simulink model "Model2"  (R2020a)
settings: Solver=ode4  StartTime=0.0  StopTime=10.0  FixedStep=0.01  RelTol=1e-3
values from neighbouring files (symbols this model uses):
  A = [0 1 0;     0 -0.875 -20;     0 0 -50]    [Zadanie1.m]    (also in Zadanie2.m = [0 1 0 0;     0 -1 0 0;     0 0 0 1;     0 0 0 -1])
  B = [0;      0;      50]    [Zadanie1.m]    (also in Zadanie2.m = [0 0;     1 0;     0 0;     0 1])
  C = eye(4)    [Zadanie2.m]
  Ff = pinv(G)    [Zadanie2.m]
  K = -Km    [Zadanie1.m]
undefined symbols (not defined in the file or in its folder): sigbuilder_block
libraries: robotcorelib x1, simulink x1
settings Model: Creator=grzyb  LastModifiedBy=grzyb

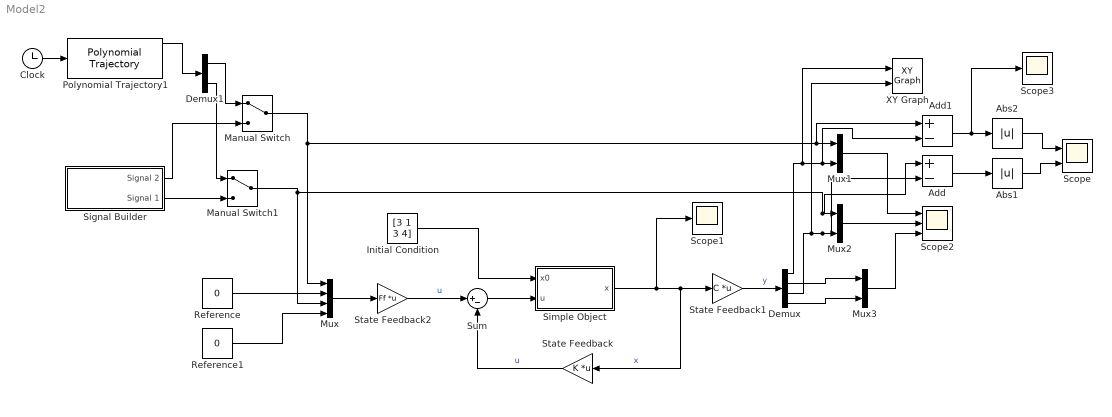
== system Model2 ==
  Abs1 : Abs
  Abs2 : Abs
  Add : Sum  Inputs=+-
  Add1 : Sum  Inputs=+-
  Clock : Clock
  Demux : Demux
  Demux1 : Demux  Outputs=2
  Initial Condition : Constant  Value=[3 1 3 4]
  Manual Switch : ManualSwitch
  Manual Switch1 : ManualSwitch
  Mux : Mux
  Mux1 : Mux  Inputs=2
  Mux2 : Mux  Inputs=2
  Mux3 : Mux  Inputs=2
  Polynomial Trajectory1 : robotcorelib/Polynomial Trajectory  WaypointSource=Internal  Waypoints=[ 0, 2, 1, 3, 0; -1, 3, 1, 4, 4 ]  TimePoints=[ 0, 2, 4, 6, 8 ]  TimeInterval=[ 1, 4 ]  Method=Cubic Polynomial  ParameterSource=Internal  VelocityBoundaryCondition=zeros( 2, 5 )  AccelerationBoundaryCondition=zeros( 2, 5 )  SimulateUsing=Interpreted execution
      settings: SourceProductBaseCode=NV,RO,RR
  Reference : Constant  Value=0
  Reference1 : Constant  Value=0
  Scope : Scope  NumInputPorts=2
  Scope1 : Scope
  Scope2 : Scope  NumInputPorts=3
  Scope3 : Scope
  Signal Builder : Subsystem  Tag=STV Subsys  LoadFcn=sigbuilder_block('load');  StartFcn=sigbuilder_block('start');  StopFcn=sigbuilder_block('stop');  ClipboardFcn=sigbuilder_block('clipboard');  mask(Sigbuilder block){tuvar=[0:10]}
      mask help: Simulink:masks:SigbuilderBlock_MD
      mask init:
      | if ~strcmp(get_param(bdroot(gcbh),'SimulationStatus'),'stopped') tuvar = sigbuilder_block('maskInit'); end
      settings: CopyFcn=sigbuilder_block('copy');  DeleteFcn=sigbuilder_block('delete');  ModelCloseFcn=sigbuilder_block('modelClose');  PreSaveFcn=sigbuilder_block('preSave');  PauseFcn=sigbuilder_block('pause');  ContinueFcn=sigbuilder_block('continue');  NameChangeFcn=sigbuilder_block('namechange');  OpenFcn=sigbuilder_block('open',[2464.8 188.4 553.2 362.4 ]);  CloseFcn=sigbuilder_block('close');
      mask Display: plot(0, 0, 100, 100,[2, 2, 32, 32, 2], [68, 8, 8, 68, 68],[32, 2], [38, 38], [32, 19, 2],[53, 60, 44], [32, 17, 17, 2],[16, 16, 31, 31]);txt = getActiveGroup(gcbh);text(2, 100, txt,'verticalAlignment', 'top');
  Simple Object : Subsystem
  State Feedback : Gain  Gain=K  Multiplication=Matrix(K*u)
  State Feedback1 : Gain  Gain=C  Multiplication=Matrix(K*u)
  State Feedback2 : Gain  Gain=Ff  Multiplication=Matrix(K*u)
  Sum : Sum  Inputs=|+-
  XY Graph : simulink/Sinks/XY Graph  xmin=-1  xmax=1  ymin=-1  ymax=1  st=-1
  wires:
  State Feedback/1 -> Sum/2  "u"
  Initial Condition/1 -> Simple Object/1(x0)
  Simple Object/1(x) -> Scope1/1, State Feedback/1, State Feedback1/1  "x"
  State Feedback1/1 -> Demux/1  "y"
  Sum/1 -> Simple Object/2(u)
  State Feedback2/1 -> Sum/1  "u"
  Mux/1 -> State Feedback2/1
  Reference/1 -> Mux/2
  Reference1/1 -> Mux/4
  Manual Switch/1 -> Mux/1, Add1/1, Mux1/1
  Mux1/1 -> Scope2/1
  Mux2/1 -> Scope2/2
  Mux3/1 -> Scope2/3
  Demux/2 -> Mux3/1
  Demux/4 -> Mux3/2
  Demux/1 -> XY Graph/1, Add1/2, Mux1/2
  Demux/3 -> XY Graph/2, Add/2, Mux2/2
  Clock/1 -> Polynomial Trajectory1/1
  Signal Builder/1(Signal 2) -> Manual Switch/2
  Signal Builder/2(Signal 1) -> Manual Switch1/2
  Polynomial Trajectory1/1 -> Demux1/1
  Demux1/1 -> Manual Switch/1
  Demux1/2 -> Manual Switch1/1
  Add/1 -> Abs1/1
  Add1/1 -> Abs2/1, Scope3/1
  Manual Switch1/1 -> Mux/3, Add/1, Mux2/1
  Abs2/1 -> Scope/1
  Abs1/1 -> Scope/2

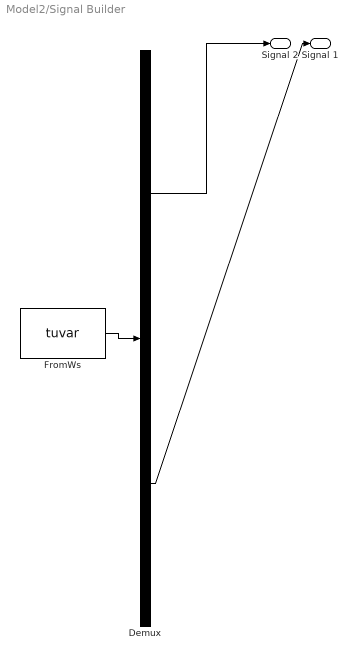
== system Model2/Signal Builder ==
  Demux : Demux  Tag=STV Demux  Outputs=2
      settings: DisplayOption=none
  FromWs : FromWorkspace  Tag=STV FromWs  VariableName=tuvar
      SigBuilderData=|
      | common.afterFinalStr = 'Extrapolate'
      | common.sampleTime = 0
      | dataSet.timeRange = [0 10]
      | dataSet.name = 'Group 1'
      | sbobj.Groups.Name = 'Group 1'
      | sbobj.Groups.Signals(1).Name = 'Signal 2'
      | sbobj.Groups.Signals(1).XData = [0 0.204081632653 0.408163265306 0.612244897959 0.816326530612 1.02040816327 1.22448979592 1.42857142857 1.63265306122 1.83673469388 2.04081632653 2.24489795918 2.44897959184 2.65306122449 2.85714285714 3.0612244898 3.26530612245 3.4693877551 3.67346938776 3.87755102041 4.08163265306 4.28571428571 4.48979591837 4.69387755102 4.89795918367 5.10204081633 5.30612244898 5.51020408163 5.71428571429 5.91836734694 6.12244897959 6.32653061224 6.5306122449 6.73469387755 6.9387755102 7.14285714286 7.34693877551 7.55102040816 7.75510204082 7.95918367347 8.16326530612 8.36734693878 8.57142857143 8.77551020408 8.97959183673 9.18367346939 9.38775510204 9.59183673469 9.79591836735 10]
      | sbobj.Groups.Signals(1).YData = [1 1.06393858084 1.12682729195 1.18763350244 1.245358776 1.29905526525 1.3478412753 1.39091574123 1.4275713815 1.45720631151 1.47933392652 1.49359089171 1.4997431081 1.49768955647 1.48746395609 1.46923421102 1.44329965319 1.4100861273 1.37013899854 1.32411419765 1.27276745061 1.21694186956 1.15755410901 1.09557931435 1.03203510999 0.96796489001 0.904420685649 0.842445890988 0.783058130441 0.727232549395 0.675885802346 0.629861001462 0.589913872702 0.556700346814 0.530765788975 0.512536043909 0.502310443525 0.5002568919 0.506409108293 0.520666073482 0.542793688492 0.572428618497 0.609084258766 0.652158724698 0.700944734754 0.754641223998 0.81236649756 0.873172708045 0.936061419158 1]
      | sbobj.Groups.Signals(2).Name = 'Signal 1'
      | sbobj.Groups.Signals(2).XData = [0 0.102040816327 0.204081632653 0.30612244898 0.408163265306 0.510204081633 0.612244897959 0.714285714286 0.816326530612 0.918367346939 1.02040816327 1.12244897959 1.22448979592 1.32653061224 1.42857142857 1.5306122449 1.63265306122 1.73469387755 1.83673469388 1.9387755102 2.04081632653 2.14285714286 2.24489795918 2.34693877551 2.44897959184 2.55102040816 2.65306122449 2.75510204082 2.85714285714 2.95918367347 3.0612244898 3.16326530612 3.26530612245 3.36734693878 3.4693877551 3.57142857143 3.67346938776 3.77551020408 3.87755102041 3.97959183673 4.08163265306 4.18367346939 4.28571428571 4.38775510204 4.48979591837 4.59183673469 4.69387755102 4.79591836735 4.89795918367 5 5.10204081633 5.20408163265 5.30612244898 5.40816326531 5.51020408163 5.61224489796 5.71428571429 5.81632653061 5.91836734694 6.02040816327 6.12244897959 6.22448979592 6.32653061224 6.42857142857 6.5306122449 6.63265306122 6.73469387755 6.83673469388 6.9387755102 7.04081632653 7.14285714286 7.24489795918 7.34693877551 7.44897959184 7.55102040816 7.65306122449 7.75510204082 7.85714285714 7.95918367347 8.0612244898 8.16326530612 8.26530612245 8.36734693878 8.4693877551 8.57142857143 8.67346938776 8.77551020408 8.87755102041 8.97959183673 9.08163265306 9.18367346939 9.28571428571 9.38775510204 9.48979591837 9.59183673469 9.69387755102 9.79591836735 9.89795918367 10]
      | sbobj.Groups.Signals(2).YData = [1 1.12787716168 1.25365458391 1.37526700488 1.490717552 1.59811053049 1.6956825506 1.78183148247 1.85514276301 1.91441262302 1.95866785304 1.98718178341 1.9994862162 1.99537911295 1.97492791218 1.93846842205 1.88659930637 1.8201722546 1.74027799708 1.64822839531 1.54553490121 1.43388373912 1.31510821802 1.1911586287 1.06407021998 0.935929780019 0.808841371299 0.684891781976 0.566116260882 0.454465098789 0.351771604692 0.259722002925 0.179827745403 0.113400693627 0.0615315779502 0.0250720878182 0.0046208870508 0.000513783799312 0.0128182165855 0.0413321469633 0.0855873769842 0.144857236995 0.218168517532 0.304317449397 0.401889469509 0.509282447996 0.624732995121 0.74634541609 0.872122838315 1 1.12787716168 1.25365458391 1.37526700488 1.490717552 1.59811053049 1.6956825506 1.78183148247 1.85514276301 1.91441262302 1.95866785304 1.98718178341 1.9994862162 1.99537911295 1.97492791218 1.93846842205 1.88659930637 1.8201722546 1.74027799708 1.64822839531 1.54553490121 1.43388373912 1.31510821802 1.1911586287 1.06407021998 0.935929780019 0.808841371299 0.684891781976 0.566116260882 0.454465098789 0.351771604692 0.259722002925 0.179827745403 0.113400693627 0.0615315779502 0.0250720878182 0.0046208870508 0.000513783799312 0.0128182165855 0.0413321469633 0.0855873769842 0.144857236995 0.218168517532 0.304317449397 0.401889469509 0.509282447996 0.624732995121 0.74634541609 0.872122838315 1]
  Signal 2 : Outport  Tag=STV Outport
  Signal 1 : Outport  Tag=STV Outport  Port=2
  wires:
  FromWs/1 -> Demux/1
  Demux/1 -> Signal 2/1
  Demux/2 -> Signal 1/1

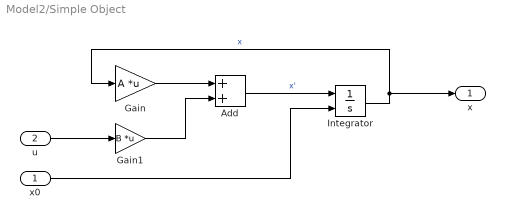
== system Model2/Simple Object ==
  x0 : Inport
  u : Inport  Port=2
  Add : Sum
  Gain : Gain  Gain=A  Multiplication=Matrix(K*u)
  Gain1 : Gain  Gain=B  Multiplication=Matrix(K*u)
  Integrator : Integrator  InitialConditionSource=external
  x : Outport
  wires:
  Integrator/1 -> x/1, Gain/1  "x"
  Add/1 -> Integrator/1  "x'"
  Gain/1 -> Add/1
  Gain1/1 -> Add/2
  u/1 -> Gain1/1
  x0/1 -> Integrator/2
